simulink model "amplificator"  (R2022b)
settings: Solver=VariableStepAuto  StartTime=0.0  StopTime=10.0  RelTol=1e-3
settings Model: Creator=fabian  LastModifiedBy=fabian

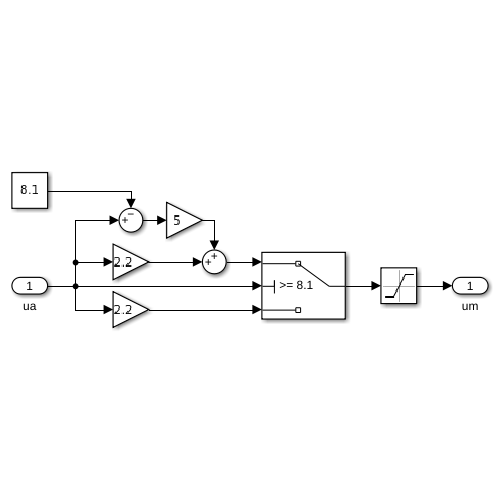
[thumbnail: Simulink's stored preview of the top-level diagram]
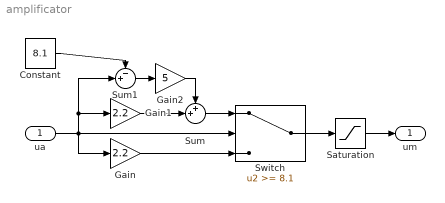
== system amplificator ==
  ua : Inport
  Constant : Constant  Value=8.1
  Gain : Gain  Gain=2.2
  Gain1 : Gain  Gain=2.2
  Gain2 : Gain  Gain=5
  Saturation : Saturate  UpperLimit=22  LowerLimit=0
  Sum : Sum  Inputs=++|
  Sum1 : Sum  Inputs=-+|
  Switch : Switch  Threshold=8.1  SaturateOnIntegerOverflow=off  InputSameDT=off
  um : Outport
  wires:
  Sum1/1 -> Gain2/1
  Sum/1 -> Switch/1
  Gain/1 -> Switch/3
  Switch/1 -> Saturation/1
  Saturation/1 -> um/1
  ua/1 -> Gain/1, Switch/2, Gain1/1, Sum1/2
  Gain1/1 -> Sum/2
  Gain2/1 -> Sum/1
  Constant/1 -> Sum1/1
